simulink model "schema_di_controllo_lineare"  (R2023b)
settings: Solver=VariableStepAuto  StartTime=0.0  StopTime=1  RelTol=1e-3
undefined symbols (not defined in the file): k, WW
libraries: cstblocks x2
settings Model: Creator=guidocarnevale  LastModifiedBy=lverc

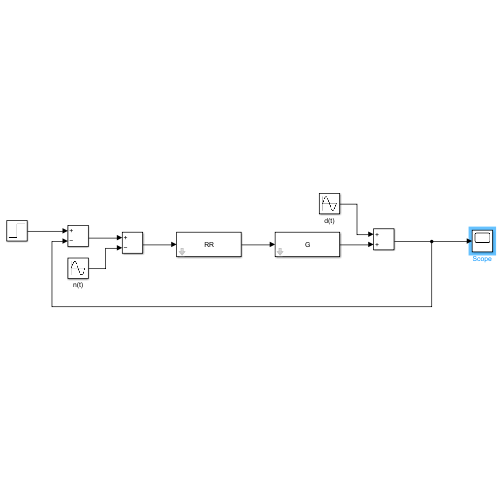
[thumbnail: Simulink's stored preview of the top-level diagram]
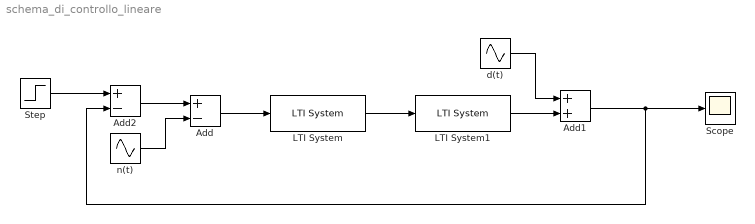
== system schema_di_controllo_lineare ==
  Add : Sum  Inputs=+-
  Add1 : Sum
  Add2 : Sum  Inputs=+-
  LTI System : cstblocks/LTI System  sys=RR  IC=[]  PadeOrder=0
  LTI System1 : cstblocks/LTI System  sys=G  IC=[]  PadeOrder=0
  Scope : Scope
  Step : Step  Time=0  After=WW  SampleTime=0
  d(t) : Sin  Amplitude=3  Frequency=0.01*k  SampleTime=0
  n(t) : Sin  Amplitude=3  Frequency=(10^5)*k  SampleTime=0
  wires:
  LTI System/1 -> LTI System1/1
  Step/1 -> Add2/1
  Add/1 -> LTI System/1
  Add2/1 -> Add/1
  n(t)/1 -> Add/2
  d(t)/1 -> Add1/1
  LTI System1/1 -> Add1/2
  Add1/1 -> Add2/2, Scope/1
